simulink library "gnss_sdr_tcp_connector_tracking_lib"  (Simulink 7.6)
settings: Solver=VariableStepDiscrete  StartTime=0.0  StopTime=10.0  RelTol=1e-3
libraries: simulink x400, instrumentlib x2, dspindex x1
(part 1 of 3)
settings Model: Creator=David Pubill  LastModifiedBy=David Pubill

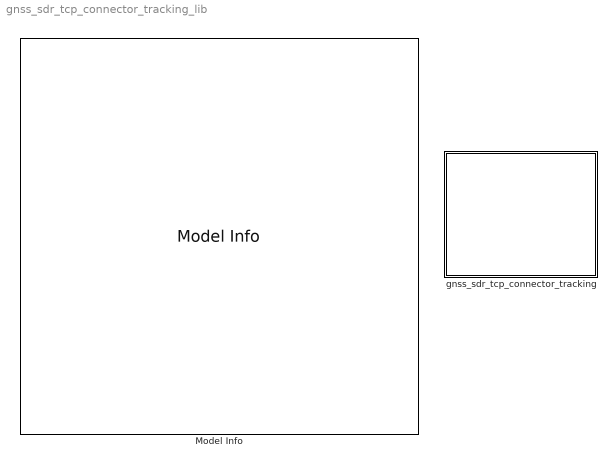
== system gnss_sdr_tcp_connector_tracking_lib ==
  Model Info : simulink/Model-Wide Utilities/Model Info  SystemSampleTime=-1  InitialBlockCM=None  BlockCM=None  Frame=on  DisplayStringWithTags=|  HorizontalTextAlignment=Left  LeftAlignmentValue=0.02  SourceBlockDiagram=gnss_sdr_tcp_connector_tracking_lib  TagMaxNumber=20
      | /*! 
      |   * \file gnss_sdr_tcp_connector_tracking_lib.mdl
      |   * \brief  gnss_sdr_tcp_connector_tracking Simulink library model. For 
      |   * further information, please read README_gnss_sdr_tcp_connector_tracking.txt
      |   *
      |   * \author David Pubill, 2012. dpubill(at)cttc.es
      |   * -------------------------------------------------------------------------
      |   *
      |   * Copyright (C) 2010-2012  (see AUTHORS file for a list of contributors)
      |   *
      |   * GNSS-SDR is a software defined Global Navigation
      |   *          Satellite Systems receiver
      |   *
      |   * This file is part of GNSS-SDR.
      |   *
      |   * GNSS-SDR is free software: you can redistribute it and/or modify
      |   * it under the terms of the GNU General Public License as published by
      |   * the Free Software Foundation, either version 3 of the License, or
      |   * at your option) any later version.
      |   *
      |   * GNSS-SDR is distributed in the hope that it will be useful,
      |   * but WITHOUT ANY WARRANTY; without even the implied warranty of
      |   * MERCHANTABILITY or FITNESS FOR A PARTICULAR PURPOSE.  See the
      |   * GNU General Public License for more details.
      |   *
      |   * You should have received a copy of the GNU General Public License
      |   * along with GNSS-SDR. If not, see <http://www.gnu.org/licenses/>.
      |   *
      |   * -------------------------------------------------------------------------
      |   */
  gnss_sdr_tcp_connector_tracking : Subsystem  AncestorBlock=simulink/User-Defined Functions/TCP_connector

== system gnss_sdr_tcp_connector_tracking_lib/gnss_sdr_tcp_connector_tracking ==
  Display : Display
  Subsystem_0 : Subsystem
  gnss_sdr_tcp_connector_tracking_receive : instrumentlib/TCP//IP Receive  DialogController=instrumentcreatedialog  DialogControllerArgs=DataTag0  Host=84.88.61.86  Port=2060  DataSize=28  EnableBlockingMode=on  Timeout=5  SampleTime=-1  DataType=uint8  ByteOrder=BigEndian
  gnss_sdr_tcp_connector_tracking_send : instrumentlib/TCP//IP Send  DialogController=instrumentcreatedialog  DialogControllerArgs=DataTag1  Host=84.88.61.86  Port=2060  EnableBlockingMode=on  Timeout=5  ByteOrder=LittleEndian
  wires:
  gnss_sdr_tcp_connector_tracking_receive/1 -> Subsystem_0/1(In)
  Subsystem_0/1(Out) -> gnss_sdr_tcp_connector_tracking_send/1, Display/1

== system gnss_sdr_tcp_connector_tracking_lib/gnss_sdr_tcp_connector_tracking/Subsystem_0 ==
  In : Inport
  Display{,1..6} (7 alike) : Display
  Multiport Selector : dspindex/Multiport Selector  rowsOrCols=Rows  idxCellArray={1,2,3,4,5,6,7,8,9,10,11,12,13,14,15,16,17,18,19,20,21,22,23,24,25,26,27,28}  idxErrMode=Clip Index
  Subsystem : Subsystem
  Subsystem1 : Subsystem
  Subsystem2 : Subsystem
  Subsystem3 : Subsystem
  Subsystem4 : Subsystem
  Subsystem5 : Subsystem
  Subsystem6 : Subsystem
  Subsystem7 : Subsystem
  Subsystem8 : Subsystem
  Vector Concatenate1 : Concatenate  NumInputs=3  Mode=Vector
  Out : Outport
  wires:
  In/1 -> Multiport Selector/1
  Vector Concatenate1/1 -> Out/1
  Multiport Selector/1 -> Subsystem/1(In1)
  Multiport Selector/2 -> Subsystem/2(In2)
  Multiport Selector/3 -> Subsystem/3(In3)
  Multiport Selector/4 -> Subsystem/4(In4)
  Multiport Selector/5 -> Subsystem1/1(In1)
  Multiport Selector/6 -> Subsystem1/2(In2)
  Multiport Selector/7 -> Subsystem1/3(In3)
  Multiport Selector/8 -> Subsystem1/4(In4)
  Multiport Selector/9 -> Subsystem2/1(In1)
  Multiport Selector/10 -> Subsystem2/2(In2)
  Multiport Selector/11 -> Subsystem2/3(In3)
  Multiport Selector/12 -> Subsystem2/4(In4)
  Multiport Selector/13 -> Subsystem3/1(In1)
  Multiport Selector/14 -> Subsystem3/2(In2)
  Multiport Selector/15 -> Subsystem3/3(In3)
  Multiport Selector/16 -> Subsystem3/4(In4)
  Subsystem/1(d_E_I) -> Subsystem7/1(d_E_I), Display/1
  Subsystem1/1(d_E_Q) -> Subsystem7/2(d_E_Q), Display1/1
  Subsystem2/1(d_L_I) -> Subsystem7/3(d_L_I), Display2/1
  Subsystem3/1(d_L_Q) -> Subsystem7/4(d_L_Q), Display3/1
  Subsystem7/1(code_error) -> Vector Concatenate1/1
  Multiport Selector/17 -> Subsystem4/1(In1)
  Multiport Selector/18 -> Subsystem4/2(In2)
  Multiport Selector/19 -> Subsystem4/3(In3)
  Multiport Selector/20 -> Subsystem4/4(In4)
  Multiport Selector/21 -> Subsystem5/1(In1)
  Multiport Selector/22 -> Subsystem5/2(In2)
  Multiport Selector/23 -> Subsystem5/3(In3)
  Multiport Selector/24 -> Subsystem5/4(In4)
  Subsystem6/1(carr_error) -> Vector Concatenate1/2
  Subsystem4/1(d_P_I) -> Subsystem6/1(d_P_I), Display4/1
  Subsystem5/1(d_P_Q) -> Subsystem6/2(d_P_Q), Display5/1
  Multiport Selector/25 -> Subsystem8/1(In1)
  Multiport Selector/26 -> Subsystem8/2(In2)
  Multiport Selector/27 -> Subsystem8/3(In3)
  Multiport Selector/28 -> Subsystem8/4(In4)
  Subsystem8/1(control_id) -> Vector Concatenate1/3, Display6/1

== system gnss_sdr_tcp_connector_tracking_lib/gnss_sdr_tcp_connector_tracking/Subsystem_0/Subsystem ==
  In1 : Inport
  In2 : Inport  Port=2
  In3 : Inport  Port=3
  In4 : Inport  Port=4
  Data Type  Conversion{1..5} (5 alike) : DataTypeConversion  OutDataTypeStr=single  SaturateOnIntegerOverflow=on  RndMeth=Zero
  hex2float : Subsystem
  d_E_I : Outport  OutputWhenDisabled=reset  InitialOutput=0
  wires:
  Data Type  Conversion5/1 -> d_E_I/1
  hex2float/1(Out1) -> Data Type  Conversion5/1
  Data Type  Conversion4/1 -> hex2float/1(In1)
  Data Type  Conversion1/1 -> hex2float/2(In2)
  Data Type  Conversion2/1 -> hex2float/3(In3)
  Data Type  Conversion3/1 -> hex2float/4(In4)
  In4/1 -> Data Type  Conversion4/1
  In3/1 -> Data Type  Conversion1/1
  In2/1 -> Data Type  Conversion2/1
  In1/1 -> Data Type  Conversion3/1

== system gnss_sdr_tcp_connector_tracking_lib/gnss_sdr_tcp_connector_tracking/Subsystem_0/Subsystem1 ==
  In1 : Inport
  In2 : Inport  Port=2
  In3 : Inport  Port=3
  In4 : Inport  Port=4
  Data Type  Conversion{1..5} (5 alike) : DataTypeConversion  OutDataTypeStr=single  SaturateOnIntegerOverflow=on  RndMeth=Zero
  hex2float : Subsystem
  d_E_Q : Outport  OutputWhenDisabled=reset  InitialOutput=0
  wires:
  In1/1 -> Data Type  Conversion3/1
  In2/1 -> Data Type  Conversion2/1
  In3/1 -> Data Type  Conversion1/1
  In4/1 -> Data Type  Conversion4/1
  Data Type  Conversion3/1 -> hex2float/4(In4)
  Data Type  Conversion2/1 -> hex2float/3(In3)
  Data Type  Conversion1/1 -> hex2float/2(In2)
  Data Type  Conversion4/1 -> hex2float/1(In1)
  hex2float/1(Out1) -> Data Type  Conversion5/1
  Data Type  Conversion5/1 -> d_E_Q/1

== system gnss_sdr_tcp_connector_tracking_lib/gnss_sdr_tcp_connector_tracking/Subsystem_0/Subsystem2 ==
  In1 : Inport
  In2 : Inport  Port=2
  In3 : Inport  Port=3
  In4 : Inport  Port=4
  Data Type  Conversion{1..5} (5 alike) : DataTypeConversion  OutDataTypeStr=single  SaturateOnIntegerOverflow=on  RndMeth=Zero
  hex2float : Subsystem
  d_L_I : Outport  OutputWhenDisabled=reset  InitialOutput=0
  wires:
  Data Type  Conversion5/1 -> d_L_I/1
  hex2float/1(Out1) -> Data Type  Conversion5/1
  Data Type  Conversion4/1 -> hex2float/1(In1)
  Data Type  Conversion1/1 -> hex2float/2(In2)
  Data Type  Conversion2/1 -> hex2float/3(In3)
  Data Type  Conversion3/1 -> hex2float/4(In4)
  In4/1 -> Data Type  Conversion4/1
  In3/1 -> Data Type  Conversion1/1
  In2/1 -> Data Type  Conversion2/1
  In1/1 -> Data Type  Conversion3/1

== system gnss_sdr_tcp_connector_tracking_lib/gnss_sdr_tcp_connector_tracking/Subsystem_0/Subsystem3 ==
  In1 : Inport
  In2 : Inport  Port=2
  In3 : Inport  Port=3
  In4 : Inport  Port=4
  Data Type  Conversion{1..5} (5 alike) : DataTypeConversion  OutDataTypeStr=single  SaturateOnIntegerOverflow=on  RndMeth=Zero
  hex2float : Subsystem
  d_L_Q : Outport  OutputWhenDisabled=reset  InitialOutput=0
  wires:
  In1/1 -> Data Type  Conversion3/1
  In2/1 -> Data Type  Conversion2/1
  In3/1 -> Data Type  Conversion1/1
  In4/1 -> Data Type  Conversion4/1
  Data Type  Conversion3/1 -> hex2float/4(In4)
  Data Type  Conversion2/1 -> hex2float/3(In3)
  Data Type  Conversion1/1 -> hex2float/2(In2)
  Data Type  Conversion4/1 -> hex2float/1(In1)
  hex2float/1(Out1) -> Data Type  Conversion5/1
  Data Type  Conversion5/1 -> d_L_Q/1

== system gnss_sdr_tcp_connector_tracking_lib/gnss_sdr_tcp_connector_tracking/Subsystem_0/Subsystem4 ==
  In1 : Inport
  In2 : Inport  Port=2
  In3 : Inport  Port=3
  In4 : Inport  Port=4
  Data Type  Conversion{1..5} (5 alike) : DataTypeConversion  OutDataTypeStr=single  SaturateOnIntegerOverflow=on  RndMeth=Zero
  hex2float : Subsystem
  d_P_I : Outport  OutputWhenDisabled=reset  InitialOutput=0
  wires:
  In1/1 -> Data Type  Conversion3/1
  In2/1 -> Data Type  Conversion2/1
  In3/1 -> Data Type  Conversion1/1
  In4/1 -> Data Type  Conversion4/1
  Data Type  Conversion3/1 -> hex2float/4(In4)
  Data Type  Conversion2/1 -> hex2float/3(In3)
  Data Type  Conversion1/1 -> hex2float/2(In2)
  Data Type  Conversion4/1 -> hex2float/1(In1)
  hex2float/1(Out1) -> Data Type  Conversion5/1
  Data Type  Conversion5/1 -> d_P_I/1

== system gnss_sdr_tcp_connector_tracking_lib/gnss_sdr_tcp_connector_tracking/Subsystem_0/Subsystem5 ==
  In1 : Inport
  In2 : Inport  Port=2
  In3 : Inport  Port=3
  In4 : Inport  Port=4
  Data Type  Conversion{1..5} (5 alike) : DataTypeConversion  OutDataTypeStr=single  SaturateOnIntegerOverflow=on  RndMeth=Zero
  hex2float : Subsystem
  d_P_Q : Outport  OutputWhenDisabled=reset  InitialOutput=0
  wires:
  Data Type  Conversion5/1 -> d_P_Q/1
  hex2float/1(Out1) -> Data Type  Conversion5/1
  Data Type  Conversion4/1 -> hex2float/1(In1)
  Data Type  Conversion1/1 -> hex2float/2(In2)
  Data Type  Conversion2/1 -> hex2float/3(In3)
  Data Type  Conversion3/1 -> hex2float/4(In4)
  In4/1 -> Data Type  Conversion4/1
  In3/1 -> Data Type  Conversion1/1
  In2/1 -> Data Type  Conversion2/1
  In1/1 -> Data Type  Conversion3/1

== system gnss_sdr_tcp_connector_tracking_lib/gnss_sdr_tcp_connector_tracking/Subsystem_0/Subsystem6 ==
  d_P_I : Inport
  d_P_Q : Inport  Port=2
  2*Pi : Constant  Value=6.283185307179586  OutDataTypeStr=double  SampleTime=-1
  Data Type  Conversion4 : DataTypeConversion  OutDataTypeStr=single  SaturateOnIntegerOverflow=on  RndMeth=Zero
  Divide1 : Product  Inputs=*/  InputSameDT=on
  Divide2 : Product  Inputs=*/  OutDataTypeStr=single  InputSameDT=on
  Trigonometric Function : Trigonometry  Operator=atan
  carr_error : Outport
  wires:
  Trigonometric Function/1 -> Divide1/1
  Divide1/1 -> carr_error/1
  d_P_I/1 -> Divide2/2
  d_P_Q/1 -> Divide2/1
  2*Pi/1 -> Data Type  Conversion4/1
  Divide2/1 -> Trigonometric Function/1
  Data Type  Conversion4/1 -> Divide1/2

== system gnss_sdr_tcp_connector_tracking_lib/gnss_sdr_tcp_connector_tracking/Subsystem_0/Subsystem7 ==
  d_E_I : Inport
  d_E_Q : Inport  Port=2
  d_L_I : Inport  Port=3
  d_L_Q : Inport  Port=4
  Ad : Sum  OutDataTypeStr=single
  Ad1 : Sum  Inputs=+-  OutDataTypeStr=single
  Ad2 : Sum  OutDataTypeStr=single
  Ad3 : Sum  OutDataTypeStr=single
  Divide : Product  Inputs=*/  InputSameDT=on
  Math Function{1..2,5..6} (4 alike) : Math  Operator=square  OutputSignalType=real  SaturateOnIntegerOverflow=on  OutDataTypeStr=Inherit: Inherit via internal rule
  Sqrt1 : Sqrt  SaturateOnIntegerOverflow=on
  Sqrt3 : Sqrt  SaturateOnIntegerOverflow=on
  code_error : Outport
  wires:
  Sqrt3/1 -> Ad1/2, Ad2/2
  Sqrt1/1 -> Ad1/1, Ad2/1
  Divide/1 -> code_error/1
  Math Function2/1 -> Ad3/2
  Math Function6/1 -> Ad3/1
  Math Function1/1 -> Ad/2
  Math Function5/1 -> Ad/1
  d_L_Q/1 -> Math Function2/1
  d_L_I/1 -> Math Function6/1
  d_E_Q/1 -> Math Function1/1
  d_E_I/1 -> Math Function5/1
  Ad/1 -> Sqrt1/1
  Ad3/1 -> Sqrt3/1
  Ad1/1 -> Divide/1
  Ad2/1 -> Divide/2

== system gnss_sdr_tcp_connector_tracking_lib/gnss_sdr_tcp_connector_tracking/Subsystem_0/Subsystem8 ==
  In1 : Inport
  In2 : Inport  Port=2
  In3 : Inport  Port=3
  In4 : Inport  Port=4
  Data Type  Conversion{1..5} (5 alike) : DataTypeConversion  OutDataTypeStr=single  SaturateOnIntegerOverflow=on  RndMeth=Zero
  hex2float : Subsystem
  control_id : Outport  OutputWhenDisabled=reset  InitialOutput=0
  wires:
  In1/1 -> Data Type  Conversion3/1
  In2/1 -> Data Type  Conversion2/1
  In3/1 -> Data Type  Conversion1/1
  In4/1 -> Data Type  Conversion4/1
  Data Type  Conversion3/1 -> hex2float/4(In4)
  Data Type  Conversion2/1 -> hex2float/3(In3)
  Data Type  Conversion1/1 -> hex2float/2(In2)
  Data Type  Conversion4/1 -> hex2float/1(In1)
  hex2float/1(Out1) -> Data Type  Conversion5/1
  Data Type  Conversion5/1 -> control_id/1

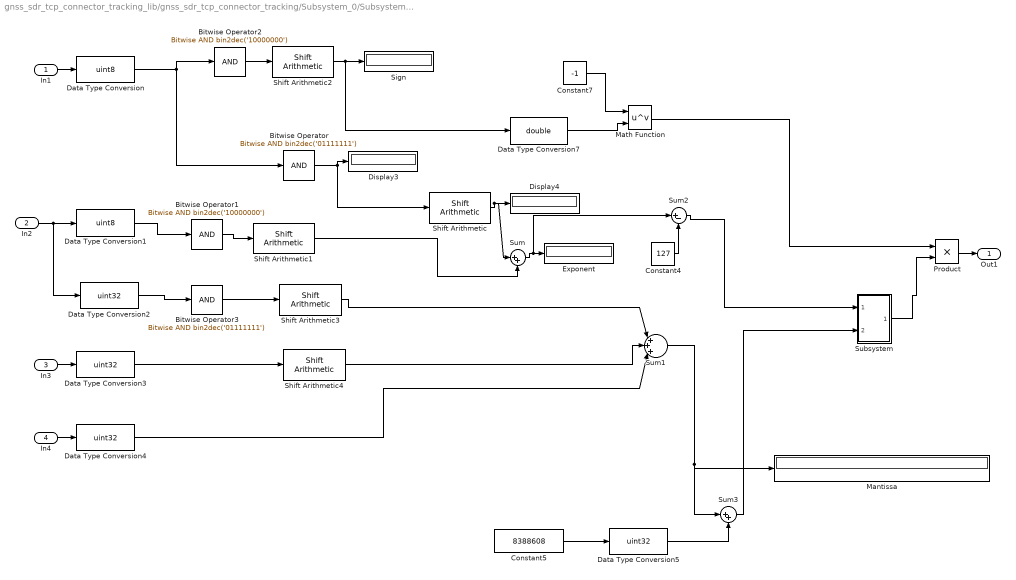
== system gnss_sdr_tcp_connector_tracking_lib/gnss_sdr_tcp_connector_tracking/Subsystem_0/Subsystem/hex2float ==
  In1 : Inport
  In2 : Inport  Port=2
  In3 : Inport  Port=3
  In4 : Inport  Port=4
  Bitwise Operator : simulink/Logic and Bit Operations/Bitwise Operator  logicop=AND  UseBitMask=on  BitMask=bin2dec('01111111')  BitMaskRealWorld=Stored Integer
  Bitwise Operator1 : simulink/Logic and Bit Operations/Bitwise Operator  logicop=AND  UseBitMask=on  BitMask=bin2dec('10000000')  BitMaskRealWorld=Stored Integer
  Bitwise Operator2 : simulink/Logic and Bit Operations/Bitwise Operator  logicop=AND  UseBitMask=on  BitMask=bin2dec('10000000')  BitMaskRealWorld=Stored Integer
  Bitwise Operator3 : simulink/Logic and Bit Operations/Bitwise Operator  logicop=AND  UseBitMask=on  BitMask=bin2dec('01111111')  BitMaskRealWorld=Stored Integer
  Constant4 : Constant  Value=127
  Constant5 : Constant  Value=8388608
  Constant7 : Constant  Value=-1
  Data Type Conversion : DataTypeConversion  OutDataTypeStr=uint8
  Data Type Conversion1 : DataTypeConversion  OutDataTypeStr=uint8
  Data Type Conversion{2..5} (4 alike) : DataTypeConversion  OutDataTypeStr=uint32
  Data Type Conversion7 : DataTypeConversion  OutDataTypeStr=double
  Display3 : Display
      settings: Format=binary (Stored Integer)
  Display4 : Display
      settings: Format=binary (Stored Integer)
  Exponent : Display
      settings: Format=binary (Stored Integer)
  Mantissa : Display
      settings: Format=binary (Stored Integer)
  Math Function : Math  Operator=pow  SaturateOnIntegerOverflow=on
  Product : Product  RndMeth=Zero
  Shift Arithmetic : simulink/Logic and Bit Operations/Shift Arithmetic  SystemSampleTime=-1  nBitShiftRight=-1  nBinPtShiftRight=0
  Shift Arithmetic1 : simulink/Logic and Bit Operations/Shift Arithmetic  SystemSampleTime=-1  nBitShiftRight=7  nBinPtShiftRight=0
  Shift Arithmetic2 : simulink/Logic and Bit Operations/Shift Arithmetic  SystemSampleTime=-1  nBitShiftRight=7  nBinPtShiftRight=0
  Shift Arithmetic3 : simulink/Logic and Bit Operations/Shift Arithmetic  SystemSampleTime=-1  nBitShiftRight=-16  nBinPtShiftRight=0
  Shift Arithmetic4 : simulink/Logic and Bit Operations/Shift Arithmetic  SystemSampleTime=-1  nBitShiftRight=-8  nBinPtShiftRight=0
  Sign : Display
      settings: Format=binary (Stored Integer)
  Subsystem : Subsystem
  Sum : Sum  Inputs=|++
  Sum1 : Sum  Inputs=|+++|
  Sum2 : Sum  Inputs=|+-
  Sum3 : Sum  Inputs=|++
  Out1 : Outport
  wires:
  Bitwise Operator/1 -> Display3/1, Shift Arithmetic/1
  Data Type Conversion/1 -> Bitwise Operator/1, Bitwise Operator2/1
  In2/1 -> Data Type Conversion2/1, Data Type Conversion1/1
  Data Type Conversion1/1 -> Bitwise Operator1/1
  Shift Arithmetic/1 -> Display4/1, Sum/1
  Bitwise Operator1/1 -> Shift Arithmetic1/1
  Shift Arithmetic1/1 -> Sum/2
  Sum/1 -> Exponent/1, Sum2/1
  Bitwise Operator2/1 -> Shift Arithmetic2/1
  Shift Arithmetic2/1 -> Sign/1, Data Type Conversion7/1
  Bitwise Operator3/1 -> Shift Arithmetic3/1
  Data Type Conversion2/1 -> Bitwise Operator3/1
  Shift Arithmetic3/1 -> Sum1/1
  Data Type Conversion3/1 -> Shift Arithmetic4/1
  Shift Arithmetic4/1 -> Sum1/2
  Data Type Conversion4/1 -> Sum1/3
  Sum1/1 -> Mantissa/1, Sum3/1
  Constant4/1 -> Sum2/2
  Sum2/1 -> Subsystem/1(In1)
  Sum3/1 -> Subsystem/2(In2)
  Constant5/1 -> Data Type Conversion5/1
  Data Type Conversion5/1 -> Sum3/2
  Subsystem/1(Out1) -> Product/2
  Constant7/1 -> Math Function/1
  Data Type Conversion7/1 -> Math Function/2
  Math Function/1 -> Product/1
  In1/1 -> Data Type Conversion/1
  Product/1 -> Out1/1
  In3/1 -> Data Type Conversion3/1
  In4/1 -> Data Type Conversion4/1

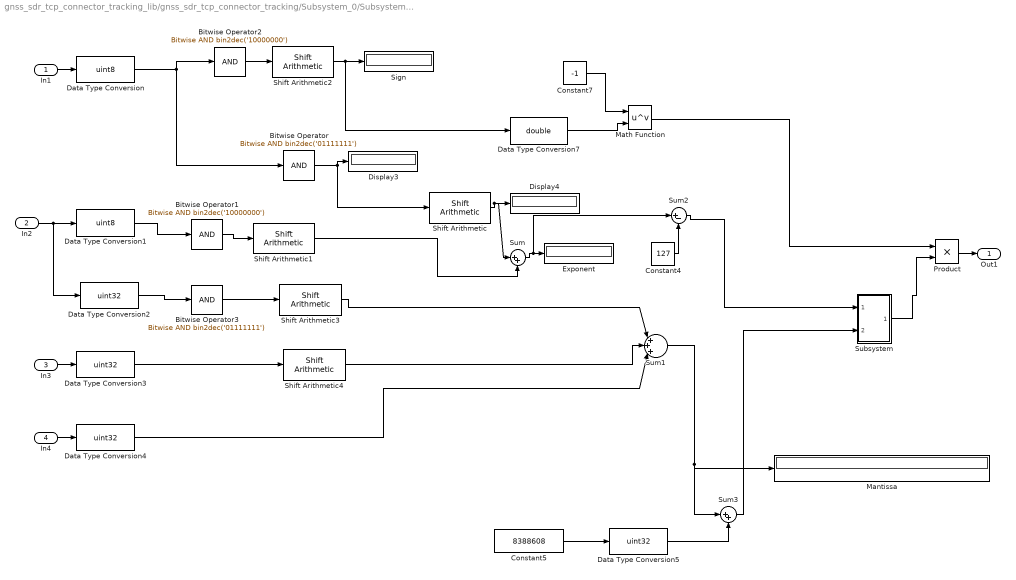
== system gnss_sdr_tcp_connector_tracking_lib/gnss_sdr_tcp_connector_tracking/Subsystem_0/Subsystem1/hex2float ==
  In1 : Inport
  In2 : Inport  Port=2
  In3 : Inport  Port=3
  In4 : Inport  Port=4
  Bitwise Operator : simulink/Logic and Bit Operations/Bitwise Operator  logicop=AND  UseBitMask=on  BitMask=bin2dec('01111111')  BitMaskRealWorld=Stored Integer
  Bitwise Operator1 : simulink/Logic and Bit Operations/Bitwise Operator  logicop=AND  UseBitMask=on  BitMask=bin2dec('10000000')  BitMaskRealWorld=Stored Integer
  Bitwise Operator2 : simulink/Logic and Bit Operations/Bitwise Operator  logicop=AND  UseBitMask=on  BitMask=bin2dec('10000000')  BitMaskRealWorld=Stored Integer
  Bitwise Operator3 : simulink/Logic and Bit Operations/Bitwise Operator  logicop=AND  UseBitMask=on  BitMask=bin2dec('01111111')  BitMaskRealWorld=Stored Integer
  Constant4 : Constant  Value=127
  Constant5 : Constant  Value=8388608
  Constant7 : Constant  Value=-1
  Data Type Conversion : DataTypeConversion  OutDataTypeStr=uint8
  Data Type Conversion1 : DataTypeConversion  OutDataTypeStr=uint8
  Data Type Conversion{2..5} (4 alike) : DataTypeConversion  OutDataTypeStr=uint32
  Data Type Conversion7 : DataTypeConversion  OutDataTypeStr=double
  Display3 : Display
      settings: Format=binary (Stored Integer)
  Display4 : Display
      settings: Format=binary (Stored Integer)
  Exponent : Display
      settings: Format=binary (Stored Integer)
  Mantissa : Display
      settings: Format=binary (Stored Integer)
  Math Function : Math  Operator=pow  SaturateOnIntegerOverflow=on
  Product : Product  RndMeth=Zero
  Shift Arithmetic : simulink/Logic and Bit Operations/Shift Arithmetic  SystemSampleTime=-1  nBitShiftRight=-1  nBinPtShiftRight=0
  Shift Arithmetic1 : simulink/Logic and Bit Operations/Shift Arithmetic  SystemSampleTime=-1  nBitShiftRight=7  nBinPtShiftRight=0
  Shift Arithmetic2 : simulink/Logic and Bit Operations/Shift Arithmetic  SystemSampleTime=-1  nBitShiftRight=7  nBinPtShiftRight=0
  Shift Arithmetic3 : simulink/Logic and Bit Operations/Shift Arithmetic  SystemSampleTime=-1  nBitShiftRight=-16  nBinPtShiftRight=0
  Shift Arithmetic4 : simulink/Logic and Bit Operations/Shift Arithmetic  SystemSampleTime=-1  nBitShiftRight=-8  nBinPtShiftRight=0
  Sign : Display
      settings: Format=binary (Stored Integer)
  Subsystem : Subsystem
  Sum : Sum  Inputs=|++
  Sum1 : Sum  Inputs=|+++|
  Sum2 : Sum  Inputs=|+-
  Sum3 : Sum  Inputs=|++
  Out1 : Outport
  wires:
  In4/1 -> Data Type Conversion4/1
  In3/1 -> Data Type Conversion3/1
  Product/1 -> Out1/1
  In1/1 -> Data Type Conversion/1
  Math Function/1 -> Product/1
  Data Type Conversion7/1 -> Math Function/2
  Constant7/1 -> Math Function/1
  Subsystem/1(Out1) -> Product/2
  Data Type Conversion5/1 -> Sum3/2
  Constant5/1 -> Data Type Conversion5/1
  Sum3/1 -> Subsystem/2(In2)
  Sum2/1 -> Subsystem/1(In1)
  Constant4/1 -> Sum2/2
  Sum1/1 -> Sum3/1, Mantissa/1
  Data Type Conversion4/1 -> Sum1/3
  Shift Arithmetic4/1 -> Sum1/2
  Data Type Conversion3/1 -> Shift Arithmetic4/1
  Shift Arithmetic3/1 -> Sum1/1
  Data Type Conversion2/1 -> Bitwise Operator3/1
  Bitwise Operator3/1 -> Shift Arithmetic3/1
  Shift Arithmetic2/1 -> Data Type Conversion7/1, Sign/1
  Bitwise Operator2/1 -> Shift Arithmetic2/1
  Sum/1 -> Sum2/1, Exponent/1
  Shift Arithmetic1/1 -> Sum/2
  Bitwise Operator1/1 -> Shift Arithmetic1/1
  Shift Arithmetic/1 -> Sum/1, Display4/1
  Data Type Conversion1/1 -> Bitwise Operator1/1
  In2/1 -> Data Type Conversion1/1, Data Type Conversion2/1
  Data Type Conversion/1 -> Bitwise Operator2/1, Bitwise Operator/1
  Bitwise Operator/1 -> Shift Arithmetic/1, Display3/1

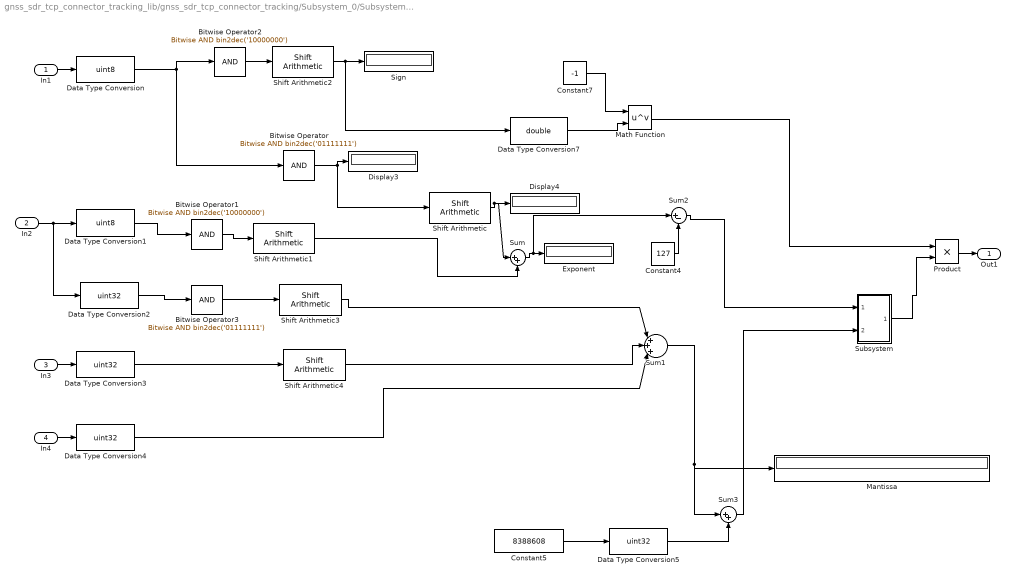
== system gnss_sdr_tcp_connector_tracking_lib/gnss_sdr_tcp_connector_tracking/Subsystem_0/Subsystem2/hex2float ==
  In1 : Inport
  In2 : Inport  Port=2
  In3 : Inport  Port=3
  In4 : Inport  Port=4
  Bitwise Operator : simulink/Logic and Bit Operations/Bitwise Operator  logicop=AND  UseBitMask=on  BitMask=bin2dec('01111111')  BitMaskRealWorld=Stored Integer
  Bitwise Operator1 : simulink/Logic and Bit Operations/Bitwise Operator  logicop=AND  UseBitMask=on  BitMask=bin2dec('10000000')  BitMaskRealWorld=Stored Integer
  Bitwise Operator2 : simulink/Logic and Bit Operations/Bitwise Operator  logicop=AND  UseBitMask=on  BitMask=bin2dec('10000000')  BitMaskRealWorld=Stored Integer
  Bitwise Operator3 : simulink/Logic and Bit Operations/Bitwise Operator  logicop=AND  UseBitMask=on  BitMask=bin2dec('01111111')  BitMaskRealWorld=Stored Integer
  Constant4 : Constant  Value=127
  Constant5 : Constant  Value=8388608
  Constant7 : Constant  Value=-1
  Data Type Conversion : DataTypeConversion  OutDataTypeStr=uint8
  Data Type Conversion1 : DataTypeConversion  OutDataTypeStr=uint8
  Data Type Conversion{2..5} (4 alike) : DataTypeConversion  OutDataTypeStr=uint32
  Data Type Conversion7 : DataTypeConversion  OutDataTypeStr=double
  Display3 : Display
      settings: Format=binary (Stored Integer)
  Display4 : Display
      settings: Format=binary (Stored Integer)
  Exponent : Display
      settings: Format=binary (Stored Integer)
  Mantissa : Display
      settings: Format=binary (Stored Integer)
  Math Function : Math  Operator=pow  SaturateOnIntegerOverflow=on
  Product : Product  RndMeth=Zero
  Shift Arithmetic : simulink/Logic and Bit Operations/Shift Arithmetic  SystemSampleTime=-1  nBitShiftRight=-1  nBinPtShiftRight=0
  Shift Arithmetic1 : simulink/Logic and Bit Operations/Shift Arithmetic  SystemSampleTime=-1  nBitShiftRight=7  nBinPtShiftRight=0
  Shift Arithmetic2 : simulink/Logic and Bit Operations/Shift Arithmetic  SystemSampleTime=-1  nBitShiftRight=7  nBinPtShiftRight=0
  Shift Arithmetic3 : simulink/Logic and Bit Operations/Shift Arithmetic  SystemSampleTime=-1  nBitShiftRight=-16  nBinPtShiftRight=0
  Shift Arithmetic4 : simulink/Logic and Bit Operations/Shift Arithmetic  SystemSampleTime=-1  nBitShiftRight=-8  nBinPtShiftRight=0
  Sign : Display
      settings: Format=binary (Stored Integer)
  Subsystem : Subsystem
  Sum : Sum  Inputs=|++
  Sum1 : Sum  Inputs=|+++|
  Sum2 : Sum  Inputs=|+-
  Sum3 : Sum  Inputs=|++
  Out1 : Outport
  wires:
  Bitwise Operator/1 -> Display3/1, Shift Arithmetic/1
  Data Type Conversion/1 -> Bitwise Operator/1, Bitwise Operator2/1
  In2/1 -> Data Type Conversion2/1, Data Type Conversion1/1
  Data Type Conversion1/1 -> Bitwise Operator1/1
  Shift Arithmetic/1 -> Display4/1, Sum/1
  Bitwise Operator1/1 -> Shift Arithmetic1/1
  Shift Arithmetic1/1 -> Sum/2
  Sum/1 -> Exponent/1, Sum2/1
  Bitwise Operator2/1 -> Shift Arithmetic2/1
  Shift Arithmetic2/1 -> Sign/1, Data Type Conversion7/1
  Bitwise Operator3/1 -> Shift Arithmetic3/1
  Data Type Conversion2/1 -> Bitwise Operator3/1
  Shift Arithmetic3/1 -> Sum1/1
  Data Type Conversion3/1 -> Shift Arithmetic4/1
  Shift Arithmetic4/1 -> Sum1/2
  Data Type Conversion4/1 -> Sum1/3
  Sum1/1 -> Mantissa/1, Sum3/1
  Constant4/1 -> Sum2/2
  Sum2/1 -> Subsystem/1(In1)
  Sum3/1 -> Subsystem/2(In2)
  Constant5/1 -> Data Type Conversion5/1
  Data Type Conversion5/1 -> Sum3/2
  Subsystem/1(Out1) -> Product/2
  Constant7/1 -> Math Function/1
  Data Type Conversion7/1 -> Math Function/2
  Math Function/1 -> Product/1
  In1/1 -> Data Type Conversion/1
  Product/1 -> Out1/1
  In3/1 -> Data Type Conversion3/1
  In4/1 -> Data Type Conversion4/1

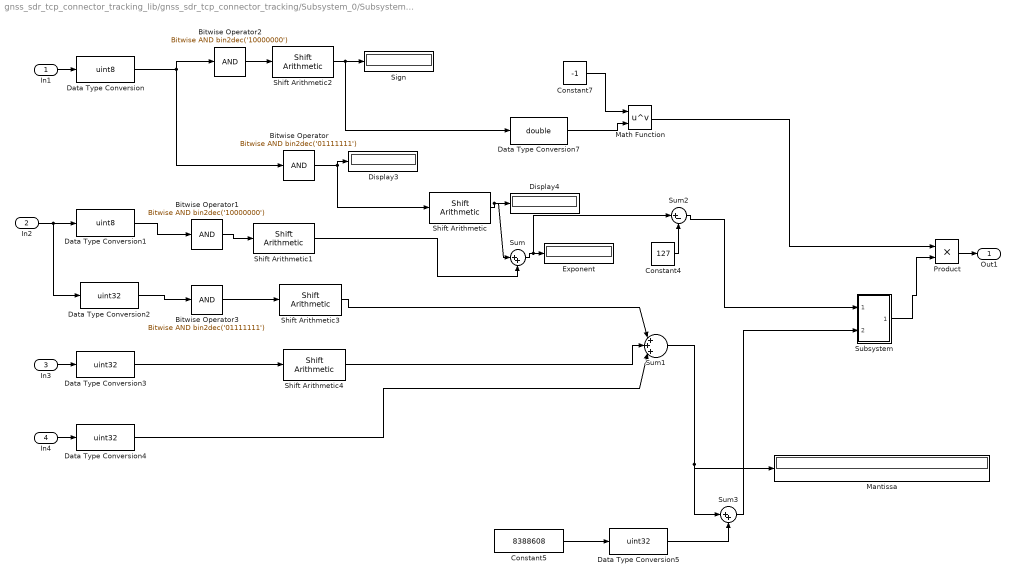
== system gnss_sdr_tcp_connector_tracking_lib/gnss_sdr_tcp_connector_tracking/Subsystem_0/Subsystem3/hex2float ==
  In1 : Inport
  In2 : Inport  Port=2
  In3 : Inport  Port=3
  In4 : Inport  Port=4
  Bitwise Operator : simulink/Logic and Bit Operations/Bitwise Operator  logicop=AND  UseBitMask=on  BitMask=bin2dec('01111111')  BitMaskRealWorld=Stored Integer
  Bitwise Operator1 : simulink/Logic and Bit Operations/Bitwise Operator  logicop=AND  UseBitMask=on  BitMask=bin2dec('10000000')  BitMaskRealWorld=Stored Integer
  Bitwise Operator2 : simulink/Logic and Bit Operations/Bitwise Operator  logicop=AND  UseBitMask=on  BitMask=bin2dec('10000000')  BitMaskRealWorld=Stored Integer
  Bitwise Operator3 : simulink/Logic and Bit Operations/Bitwise Operator  logicop=AND  UseBitMask=on  BitMask=bin2dec('01111111')  BitMaskRealWorld=Stored Integer
  Constant4 : Constant  Value=127
  Constant5 : Constant  Value=8388608
  Constant7 : Constant  Value=-1
  Data Type Conversion : DataTypeConversion  OutDataTypeStr=uint8
  Data Type Conversion1 : DataTypeConversion  OutDataTypeStr=uint8
  Data Type Conversion{2..5} (4 alike) : DataTypeConversion  OutDataTypeStr=uint32
  Data Type Conversion7 : DataTypeConversion  OutDataTypeStr=double
  Display3 : Display
      settings: Format=binary (Stored Integer)
  Display4 : Display
      settings: Format=binary (Stored Integer)
  Exponent : Display
      settings: Format=binary (Stored Integer)
  Mantissa : Display
      settings: Format=binary (Stored Integer)
  Math Function : Math  Operator=pow  SaturateOnIntegerOverflow=on
  Product : Product  RndMeth=Zero
  Shift Arithmetic : simulink/Logic and Bit Operations/Shift Arithmetic  SystemSampleTime=-1  nBitShiftRight=-1  nBinPtShiftRight=0
  Shift Arithmetic1 : simulink/Logic and Bit Operations/Shift Arithmetic  SystemSampleTime=-1  nBitShiftRight=7  nBinPtShiftRight=0
  Shift Arithmetic2 : simulink/Logic and Bit Operations/Shift Arithmetic  SystemSampleTime=-1  nBitShiftRight=7  nBinPtShiftRight=0
  Shift Arithmetic3 : simulink/Logic and Bit Operations/Shift Arithmetic  SystemSampleTime=-1  nBitShiftRight=-16  nBinPtShiftRight=0
  Shift Arithmetic4 : simulink/Logic and Bit Operations/Shift Arithmetic  SystemSampleTime=-1  nBitShiftRight=-8  nBinPtShiftRight=0
  Sign : Display
      settings: Format=binary (Stored Integer)
  Subsystem : Subsystem
  Sum : Sum  Inputs=|++
  Sum1 : Sum  Inputs=|+++|
  Sum2 : Sum  Inputs=|+-
  Sum3 : Sum  Inputs=|++
  Out1 : Outport
  wires:
  In4/1 -> Data Type Conversion4/1
  In3/1 -> Data Type Conversion3/1
  Product/1 -> Out1/1
  In1/1 -> Data Type Conversion/1
  Math Function/1 -> Product/1
  Data Type Conversion7/1 -> Math Function/2
  Constant7/1 -> Math Function/1
  Subsystem/1(Out1) -> Product/2
  Data Type Conversion5/1 -> Sum3/2
  Constant5/1 -> Data Type Conversion5/1
  Sum3/1 -> Subsystem/2(In2)
  Sum2/1 -> Subsystem/1(In1)
  Constant4/1 -> Sum2/2
  Sum1/1 -> Sum3/1, Mantissa/1
  Data Type Conversion4/1 -> Sum1/3
  Shift Arithmetic4/1 -> Sum1/2
  Data Type Conversion3/1 -> Shift Arithmetic4/1
  Shift Arithmetic3/1 -> Sum1/1
  Data Type Conversion2/1 -> Bitwise Operator3/1
  Bitwise Operator3/1 -> Shift Arithmetic3/1
  Shift Arithmetic2/1 -> Data Type Conversion7/1, Sign/1
  Bitwise Operator2/1 -> Shift Arithmetic2/1
  Sum/1 -> Sum2/1, Exponent/1
  Shift Arithmetic1/1 -> Sum/2
  Bitwise Operator1/1 -> Shift Arithmetic1/1
  Shift Arithmetic/1 -> Sum/1, Display4/1
  Data Type Conversion1/1 -> Bitwise Operator1/1
  In2/1 -> Data Type Conversion1/1, Data Type Conversion2/1
  Data Type Conversion/1 -> Bitwise Operator2/1, Bitwise Operator/1
  Bitwise Operator/1 -> Shift Arithmetic/1, Display3/1

== system gnss_sdr_tcp_connector_tracking_lib/gnss_sdr_tcp_connector_tracking/Subsystem_0/Subsystem4/hex2float ==
  In1 : Inport
  In2 : Inport  Port=2
  In3 : Inport  Port=3
  In4 : Inport  Port=4
  Bitwise Operator : simulink/Logic and Bit Operations/Bitwise Operator  logicop=AND  UseBitMask=on  BitMask=bin2dec('01111111')  BitMaskRealWorld=Stored Integer
  Bitwise Operator1 : simulink/Logic and Bit Operations/Bitwise Operator  logicop=AND  UseBitMask=on  BitMask=bin2dec('10000000')  BitMaskRealWorld=Stored Integer
  Bitwise Operator2 : simulink/Logic and Bit Operations/Bitwise Operator  logicop=AND  UseBitMask=on  BitMask=bin2dec('10000000')  BitMaskRealWorld=Stored Integer
  Bitwise Operator3 : simulink/Logic and Bit Operations/Bitwise Operator  logicop=AND  UseBitMask=on  BitMask=bin2dec('01111111')  BitMaskRealWorld=Stored Integer
  Constant4 : Constant  Value=127
  Constant5 : Constant  Value=8388608
  Constant7 : Constant  Value=-1
  Data Type Conversion : DataTypeConversion  OutDataTypeStr=uint8
  Data Type Conversion1 : DataTypeConversion  OutDataTypeStr=uint8
  Data Type Conversion{2..5} (4 alike) : DataTypeConversion  OutDataTypeStr=uint32
  Data Type Conversion7 : DataTypeConversion  OutDataTypeStr=double
  Display3 : Display
      settings: Format=binary (Stored Integer)
  Display4 : Display
      settings: Format=binary (Stored Integer)
  Exponent : Display
      settings: Format=binary (Stored Integer)
  Mantissa : Display
      settings: Format=binary (Stored Integer)
  Math Function : Math  Operator=pow  SaturateOnIntegerOverflow=on
  Product : Product  RndMeth=Zero
  Shift Arithmetic : simulink/Logic and Bit Operations/Shift Arithmetic  SystemSampleTime=-1  nBitShiftRight=-1  nBinPtShiftRight=0
  Shift Arithmetic1 : simulink/Logic and Bit Operations/Shift Arithmetic  SystemSampleTime=-1  nBitShiftRight=7  nBinPtShiftRight=0
  Shift Arithmetic2 : simulink/Logic and Bit Operations/Shift Arithmetic  SystemSampleTime=-1  nBitShiftRight=7  nBinPtShiftRight=0
  Shift Arithmetic3 : simulink/Logic and Bit Operations/Shift Arithmetic  SystemSampleTime=-1  nBitShiftRight=-16  nBinPtShiftRight=0
  Shift Arithmetic4 : simulink/Logic and Bit Operations/Shift Arithmetic  SystemSampleTime=-1  nBitShiftRight=-8  nBinPtShiftRight=0
  Sign : Display
      settings: Format=binary (Stored Integer)
  Subsystem : Subsystem
  Sum : Sum  Inputs=|++
  Sum1 : Sum  Inputs=|+++|
  Sum2 : Sum  Inputs=|+-
  Sum3 : Sum  Inputs=|++
  Out1 : Outport
  wires:
  In4/1 -> Data Type Conversion4/1
  In3/1 -> Data Type Conversion3/1
  Product/1 -> Out1/1
  In1/1 -> Data Type Conversion/1
  Math Function/1 -> Product/1
  Data Type Conversion7/1 -> Math Function/2
  Constant7/1 -> Math Function/1
  Subsystem/1(Out1) -> Product/2
  Data Type Conversion5/1 -> Sum3/2
  Constant5/1 -> Data Type Conversion5/1
  Sum3/1 -> Subsystem/2(In2)
  Sum2/1 -> Subsystem/1(In1)
  Constant4/1 -> Sum2/2
  Sum1/1 -> Sum3/1, Mantissa/1
  Data Type Conversion4/1 -> Sum1/3
  Shift Arithmetic4/1 -> Sum1/2
  Data Type Conversion3/1 -> Shift Arithmetic4/1
  Shift Arithmetic3/1 -> Sum1/1
  Data Type Conversion2/1 -> Bitwise Operator3/1
  Bitwise Operator3/1 -> Shift Arithmetic3/1
  Shift Arithmetic2/1 -> Data Type Conversion7/1, Sign/1
  Bitwise Operator2/1 -> Shift Arithmetic2/1
  Sum/1 -> Sum2/1, Exponent/1
  Shift Arithmetic1/1 -> Sum/2
  Bitwise Operator1/1 -> Shift Arithmetic1/1
  Shift Arithmetic/1 -> Sum/1, Display4/1
  Data Type Conversion1/1 -> Bitwise Operator1/1
  In2/1 -> Data Type Conversion1/1, Data Type Conversion2/1
  Data Type Conversion/1 -> Bitwise Operator2/1, Bitwise Operator/1
  Bitwise Operator/1 -> Shift Arithmetic/1, Display3/1

== system gnss_sdr_tcp_connector_tracking_lib/gnss_sdr_tcp_connector_tracking/Subsystem_0/Subsystem5/hex2float ==
  In1 : Inport
  In2 : Inport  Port=2
  In3 : Inport  Port=3
  In4 : Inport  Port=4
  Bitwise Operator : simulink/Logic and Bit Operations/Bitwise Operator  logicop=AND  UseBitMask=on  BitMask=bin2dec('01111111')  BitMaskRealWorld=Stored Integer
  Bitwise Operator1 : simulink/Logic and Bit Operations/Bitwise Operator  logicop=AND  UseBitMask=on  BitMask=bin2dec('10000000')  BitMaskRealWorld=Stored Integer
  Bitwise Operator2 : simulink/Logic and Bit Operations/Bitwise Operator  logicop=AND  UseBitMask=on  BitMask=bin2dec('10000000')  BitMaskRealWorld=Stored Integer
  Bitwise Operator3 : simulink/Logic and Bit Operations/Bitwise Operator  logicop=AND  UseBitMask=on  BitMask=bin2dec('01111111')  BitMaskRealWorld=Stored Integer
  Constant4 : Constant  Value=127
  Constant5 : Constant  Value=8388608
  Constant7 : Constant  Value=-1
  Data Type Conversion : DataTypeConversion  OutDataTypeStr=uint8
  Data Type Conversion1 : DataTypeConversion  OutDataTypeStr=uint8
  Data Type Conversion{2..5} (4 alike) : DataTypeConversion  OutDataTypeStr=uint32
  Data Type Conversion7 : DataTypeConversion  OutDataTypeStr=double
  Display3 : Display
      settings: Format=binary (Stored Integer)
  Display4 : Display
      settings: Format=binary (Stored Integer)
  Exponent : Display
      settings: Format=binary (Stored Integer)
  Mantissa : Display
      settings: Format=binary (Stored Integer)
  Math Function : Math  Operator=pow  SaturateOnIntegerOverflow=on
  Product : Product  RndMeth=Zero
  Shift Arithmetic : simulink/Logic and Bit Operations/Shift Arithmetic  SystemSampleTime=-1  nBitShiftRight=-1  nBinPtShiftRight=0
  Shift Arithmetic1 : simulink/Logic and Bit Operations/Shift Arithmetic  SystemSampleTime=-1  nBitShiftRight=7  nBinPtShiftRight=0
  Shift Arithmetic2 : simulink/Logic and Bit Operations/Shift Arithmetic  SystemSampleTime=-1  nBitShiftRight=7  nBinPtShiftRight=0
  Shift Arithmetic3 : simulink/Logic and Bit Operations/Shift Arithmetic  SystemSampleTime=-1  nBitShiftRight=-16  nBinPtShiftRight=0
  Shift Arithmetic4 : simulink/Logic and Bit Operations/Shift Arithmetic  SystemSampleTime=-1  nBitShiftRight=-8  nBinPtShiftRight=0
  Sign : Display
      settings: Format=binary (Stored Integer)
  Subsystem : Subsystem
  Sum : Sum  Inputs=|++
  Sum1 : Sum  Inputs=|+++|
  Sum2 : Sum  Inputs=|+-
  Sum3 : Sum  Inputs=|++
  Out1 : Outport
  wires:
  Bitwise Operator/1 -> Display3/1, Shift Arithmetic/1
  Data Type Conversion/1 -> Bitwise Operator/1, Bitwise Operator2/1
  In2/1 -> Data Type Conversion2/1, Data Type Conversion1/1
  Data Type Conversion1/1 -> Bitwise Operator1/1
  Shift Arithmetic/1 -> Display4/1, Sum/1
  Bitwise Operator1/1 -> Shift Arithmetic1/1
  Shift Arithmetic1/1 -> Sum/2
  Sum/1 -> Exponent/1, Sum2/1
  Bitwise Operator2/1 -> Shift Arithmetic2/1
  Shift Arithmetic2/1 -> Sign/1, Data Type Conversion7/1
  Bitwise Operator3/1 -> Shift Arithmetic3/1
  Data Type Conversion2/1 -> Bitwise Operator3/1
  Shift Arithmetic3/1 -> Sum1/1
  Data Type Conversion3/1 -> Shift Arithmetic4/1
  Shift Arithmetic4/1 -> Sum1/2
  Data Type Conversion4/1 -> Sum1/3
  Sum1/1 -> Mantissa/1, Sum3/1
  Constant4/1 -> Sum2/2
  Sum2/1 -> Subsystem/1(In1)
  Sum3/1 -> Subsystem/2(In2)
  Constant5/1 -> Data Type Conversion5/1
  Data Type Conversion5/1 -> Sum3/2
  Subsystem/1(Out1) -> Product/2
  Constant7/1 -> Math Function/1
  Data Type Conversion7/1 -> Math Function/2
  Math Function/1 -> Product/1
  In1/1 -> Data Type Conversion/1
  Product/1 -> Out1/1
  In3/1 -> Data Type Conversion3/1
  In4/1 -> Data Type Conversion4/1

== system gnss_sdr_tcp_connector_tracking_lib/gnss_sdr_tcp_connector_tracking/Subsystem_0/Subsystem8/hex2float ==
  In1 : Inport
  In2 : Inport  Port=2
  In3 : Inport  Port=3
  In4 : Inport  Port=4
  Bitwise Operator : simulink/Logic and Bit Operations/Bitwise Operator  logicop=AND  UseBitMask=on  BitMask=bin2dec('01111111')  BitMaskRealWorld=Stored Integer
  Bitwise Operator1 : simulink/Logic and Bit Operations/Bitwise Operator  logicop=AND  UseBitMask=on  BitMask=bin2dec('10000000')  BitMaskRealWorld=Stored Integer
  Bitwise Operator2 : simulink/Logic and Bit Operations/Bitwise Operator  logicop=AND  UseBitMask=on  BitMask=bin2dec('10000000')  BitMaskRealWorld=Stored Integer
  Bitwise Operator3 : simulink/Logic and Bit Operations/Bitwise Operator  logicop=AND  UseBitMask=on  BitMask=bin2dec('01111111')  BitMaskRealWorld=Stored Integer
  Constant4 : Constant  Value=127
  Constant5 : Constant  Value=8388608
  Constant7 : Constant  Value=-1
  Data Type Conversion : DataTypeConversion  OutDataTypeStr=uint8
  Data Type Conversion1 : DataTypeConversion  OutDataTypeStr=uint8
  Data Type Conversion{2..5} (4 alike) : DataTypeConversion  OutDataTypeStr=uint32
  Data Type Conversion7 : DataTypeConversion  OutDataTypeStr=double
  Display3 : Display
      settings: Format=binary (Stored Integer)
  Display4 : Display
      settings: Format=binary (Stored Integer)
  Exponent : Display
      settings: Format=binary (Stored Integer)
  Mantissa : Display
      settings: Format=binary (Stored Integer)
  Math Function : Math  Operator=pow  SaturateOnIntegerOverflow=on
  Product : Product  RndMeth=Zero
  Shift Arithmetic : simulink/Logic and Bit Operations/Shift Arithmetic  SystemSampleTime=-1  nBitShiftRight=-1  nBinPtShiftRight=0
  Shift Arithmetic1 : simulink/Logic and Bit Operations/Shift Arithmetic  SystemSampleTime=-1  nBitShiftRight=7  nBinPtShiftRight=0
  Shift Arithmetic2 : simulink/Logic and Bit Operations/Shift Arithmetic  SystemSampleTime=-1  nBitShiftRight=7  nBinPtShiftRight=0
  Shift Arithmetic3 : simulink/Logic and Bit Operations/Shift Arithmetic  SystemSampleTime=-1  nBitShiftRight=-16  nBinPtShiftRight=0
  Shift Arithmetic4 : simulink/Logic and Bit Operations/Shift Arithmetic  SystemSampleTime=-1  nBitShiftRight=-8  nBinPtShiftRight=0
  Sign : Display
      settings: Format=binary (Stored Integer)
  Subsystem : Subsystem
  Sum : Sum  Inputs=|++
  Sum1 : Sum  Inputs=|+++|
  Sum2 : Sum  Inputs=|+-
  Sum3 : Sum  Inputs=|++
  Out1 : Outport
  wires:
  In4/1 -> Data Type Conversion4/1
  In3/1 -> Data Type Conversion3/1
  Product/1 -> Out1/1
  In1/1 -> Data Type Conversion/1
  Math Function/1 -> Product/1
  Data Type Conversion7/1 -> Math Function/2
  Constant7/1 -> Math Function/1
  Subsystem/1(Out1) -> Product/2
  Data Type Conversion5/1 -> Sum3/2
  Constant5/1 -> Data Type Conversion5/1
  Sum3/1 -> Subsystem/2(In2)
  Sum2/1 -> Subsystem/1(In1)
  Constant4/1 -> Sum2/2
  Sum1/1 -> Sum3/1, Mantissa/1
  Data Type Conversion4/1 -> Sum1/3
  Shift Arithmetic4/1 -> Sum1/2
  Data Type Conversion3/1 -> Shift Arithmetic4/1
  Shift Arithmetic3/1 -> Sum1/1
  Data Type Conversion2/1 -> Bitwise Operator3/1
  Bitwise Operator3/1 -> Shift Arithmetic3/1
  Shift Arithmetic2/1 -> Data Type Conversion7/1, Sign/1
  Bitwise Operator2/1 -> Shift Arithmetic2/1
  Sum/1 -> Sum2/1, Exponent/1
  Shift Arithmetic1/1 -> Sum/2
  Bitwise Operator1/1 -> Shift Arithmetic1/1
  Shift Arithmetic/1 -> Sum/1, Display4/1
  Data Type Conversion1/1 -> Bitwise Operator1/1
  In2/1 -> Data Type Conversion1/1, Data Type Conversion2/1
  Data Type Conversion/1 -> Bitwise Operator2/1, Bitwise Operator/1
  Bitwise Operator/1 -> Shift Arithmetic/1, Display3/1
